simulink model "APPLookUpTable"  (R2022b)
settings: Solver=VariableStepAuto  StartTime=0.0  StopTime=10.0  RelTol=1e-3
libraries: simulink x1
settings Model: Creator=ahmed  LastModifiedBy=ahmed
settings DataIOCC: LoadExternalInput=on

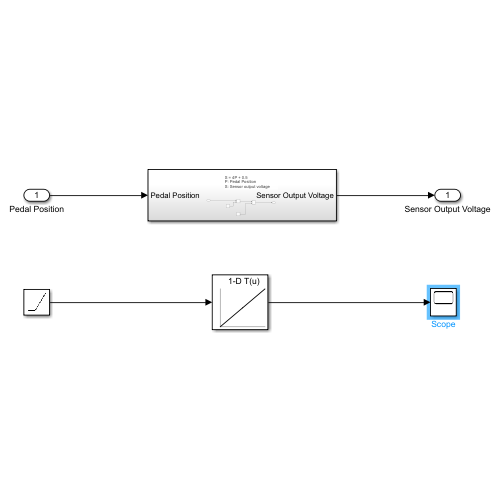
[thumbnail: Simulink's stored preview of the top-level diagram]
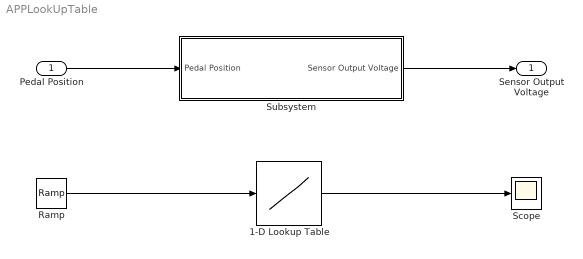
== system APPLookUpTable ==
  Pedal Position : Inport
  1-D Lookup Table : Lookup_n-D  NumberOfTableDimensions=1  BreakpointsForDimension1=[0 0.5 1]  Table=[0.5 2.5 4.5]  InternalRulePriority=Speed  RndMeth=Simplest
  Ramp : simulink/Sources/Ramp  slope=1  start=0  InitialOutput=0
  Scope : Scope
  Subsystem : Subsystem
  Sensor Output Voltage : Outport
  wires:
  Pedal Position/1 -> Subsystem/1(Pedal Position)
  Subsystem/1(Sensor Output Voltage) -> Sensor Output Voltage/1
  1-D Lookup Table/1 -> Scope/1
  Ramp/1 -> 1-D Lookup Table/1

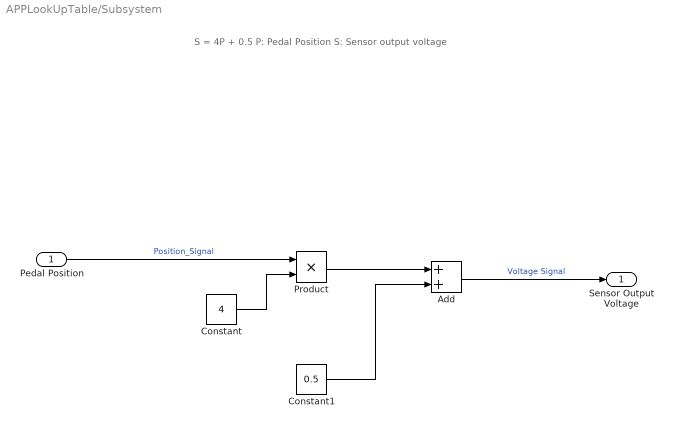
== system APPLookUpTable/Subsystem ==
  note: S = 4P + 0.5
      | P: Pedal Position
      | S: Sensor output voltage
  Pedal Position : Inport
  Add : Sum
  Constant : Constant  Value=4
  Constant1 : Constant  Value=0.5
  Product : Product
  Sensor Output Voltage : Outport
  wires:
  Constant/1 -> Product/2
  Product/1 -> Add/1
  Pedal Position/1 -> Product/1  "Position_Signal"
  Add/1 -> Sensor Output Voltage/1  "Voltage Signal"
  Constant1/1 -> Add/2
